simulink model "sys2"  (R2019a)
settings: Solver=FixedStepAuto  StartTime=0.0  StopTime=100.0  FixedStep=0.01  RelTol=1e-3
InitFcn:
  | sys2Mec
values from neighbouring files (symbols this model uses):
  x0 = x    [sys2Mec.m]
libraries: simulink x1
settings Model: Creator=alfyhack  LastModifiedBy=alfyhack

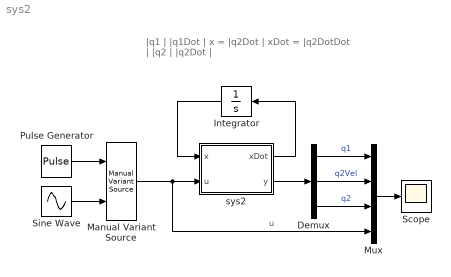
== system sys2 ==
  note: |q1		|      		 	|q1Dot   		|
      | x = |q2Dot 	|	 xDot = 	|q2DotDot	|
      |       |q2       	|        		|q2Dot  		|
  Demux : Demux  Outputs=3
  Integrator : Integrator  InitialCondition=x0
  Manual Variant Source : simulink/Signal Routing/Manual Variant Source  NumChoices=2  LabelModeActiveChoice=V_1
      settings: SourceProductName=Simulink
  Mux : Mux
  Pulse Generator : DiscretePulseGenerator  PulseType=Time based  Period=10  PulseWidth=10
  Scope : Scope
  Sine Wave : Sin  SampleTime=0
  sys2 : MATLAB Function  TreatAsAtomicUnit=on
  wires:
  sys2/1(xDot) -> Integrator/1
  Integrator/1 -> sys2/1(x)
  Pulse Generator/1 -> Manual Variant Source/1
  Sine Wave/1 -> Manual Variant Source/2
  Manual Variant Source/1 -> Mux/4, sys2/2(u)  "u"
  sys2/2(y) -> Demux/1
  Mux/1 -> Scope/1
  Demux/3 -> Mux/3  "q2"
  Demux/2 -> Mux/2  "q2Vel"
  Demux/1 -> Mux/1  "q1"

== matlab function sys2/sys2 ==
  data: x input; u input; xDot output; y output
function [xDot,y] = sys2Diff(x,u)
%SYS2DIF Summary of this function goes here
%     |q1   |        |q1Dot   |
% x = |q2Dot| xDot = |q2DotDot|
%     |q2   |        |q2Dot   |

D=1;
M=1;
K=1;
xDot = zeros(3,1);

xDot(1) = -K/M*x(1)+x(2);
xDot(2) = -K/M*x(1) + u/M;
xDot(3) = x(2);
y=x;
end
